simulink model "prelab2_step_resp"  (R2018b)
settings: Solver=FixedStepAuto  StartTime=0.0  StopTime=0.75  FixedStep=0.001  RelTol=1e-3
values from neighbouring files (symbols this model uses):
  plnt_poles = [0.0003642065 0.0778413 1]    [matlab.mat]    (also in prelab2.m)
  plnt_zeros = [-0.13361655 26.7233]    [matlab.mat]    (also in prelab2.m)
  z1 = -23.5    [matlab.mat]    (also in prelab2.m = int(min_index))
  z2 = -11.75    [matlab.mat]    (also in prelab2.m = z1/2)
  z3 = -7.83333333333    [matlab.mat]    (also in prelab2.m = z1/3)
settings Model: Creator=Dell  LastModifiedBy=Dell

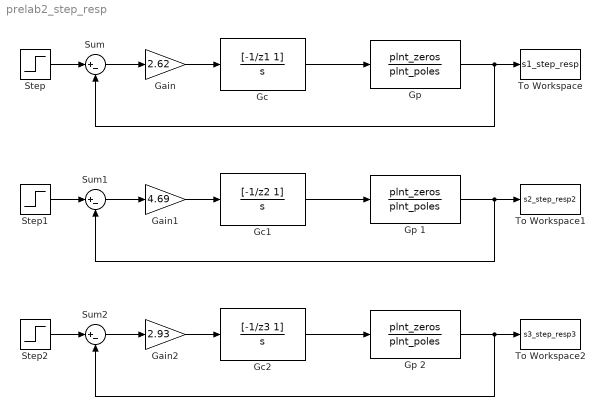
== system prelab2_step_resp ==
  Gain : Gain  Gain=2.62
  Gain1 : Gain  Gain=4.69
  Gain2 : Gain  Gain=2.93
  Gc : TransferFcn  Numerator=[-1/z1 1]  Denominator=[1 0]
  Gc1 : TransferFcn  Numerator=[-1/z2 1]  Denominator=[1 0]
  Gc2 : TransferFcn  Numerator=[-1/z3 1]  Denominator=[1 0]
  "Gp " : TransferFcn  Numerator=plnt_zeros  Denominator=plnt_poles
  Gp 1 : TransferFcn  Numerator=plnt_zeros  Denominator=plnt_poles
  Gp 2 : TransferFcn  Numerator=plnt_zeros  Denominator=plnt_poles
  Step : Step  Time=0  After=10  SampleTime=0
  Step1 : Step  Time=0  After=10  SampleTime=0
  Step2 : Step  Time=0  After=10  SampleTime=0
  Sum : Sum  Inputs=|+-
  Sum1 : Sum  Inputs=|+-
  Sum2 : Sum  Inputs=|+-
  To Workspace : ToWorkspace  VariableName=s1_step_resp  SaveFormat=Timeseries  SampleTime=-1
  To Workspace1 : ToWorkspace  VariableName=s2_step_resp2  SaveFormat=Timeseries  SampleTime=-1
  To Workspace2 : ToWorkspace  VariableName=s3_step_resp3  SaveFormat=Timeseries  SampleTime=-1
  wires:
  Gc/1 -> "Gp "/1
  Step/1 -> Sum/1
  Sum/1 -> Gain/1
  Gain/1 -> Gc/1
  "Gp "/1 -> Sum/2, To Workspace/1
  Gp 1/1 -> Sum1/2, To Workspace1/1
  Step1/1 -> Sum1/1
  Sum1/1 -> Gain1/1
  Gc1/1 -> Gp 1/1
  Gain1/1 -> Gc1/1
  Gp 2/1 -> Sum2/2, To Workspace2/1
  Step2/1 -> Sum2/1
  Sum2/1 -> Gain2/1
  Gc2/1 -> Gp 2/1
  Gain2/1 -> Gc2/1
